simulink model "Signal_Generate_PRN1"  (Simulink 7.3)
settings: Solver=ode45  StartTime=0.0  StopTime=10.0  RelTol=1e-3
values from neighbouring files (symbols this model uses):
  prn = [1 1 1 1 1 1 1 1 1 1 1 1 ... (32736 elements, 32x1023)]    [prn_codes.mat]
libraries: simulink x3, dspswit3 x3, commsynccomp2 x2
settings Model: Creator=xiruizhifu  LastModifiedBy=xiruizhifu
settings SimEventsCC: propDiagAttribOutput=1  propDiagFcnCallOutput=1  propDiagStatOutput=0

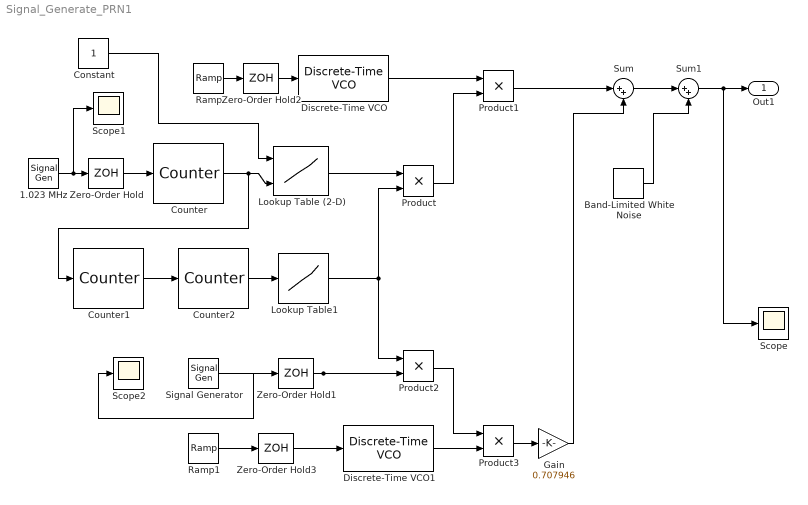
== system Signal_Generate_PRN1 ==
  1.023 MHz : SignalGenerator  WaveForm=square  Frequency=1023000
  Band-Limited White Noise : simulink/Sources/Band-Limited White Noise  SystemSampleTime=-1  Cov=[0.1]  Ts=0.1  seed=[23341]
  Constant : Constant  OutDataType=fixdt(1, 16)  OutScaling=2^0
  Counter : dspswit3/Counter  Direction=Up  CountEvent=Falling edge  CounterSize=User defined  MaxCount=1022  InitialCount=233  Output=Count  HitValue=32  ResetInput=off  SamplesPerFrame=1  Ts=1  CntDtype=double  HitDtype=Logical
  Counter1 : dspswit3/Counter  Direction=Up  CountEvent=Falling edge  CounterSize=User defined  MaxCount=20  InitialCount=0  Output=Count  HitValue=32  ResetInput=off  SamplesPerFrame=1  Ts=1  CntDtype=double  HitDtype=Logical
  Counter2 : dspswit3/Counter  Direction=Up  CountEvent=Falling edge  CounterSize=User defined  MaxCount=1500  InitialCount=0  Output=Count  HitValue=32  ResetInput=off  SamplesPerFrame=1  Ts=1  CntDtype=double  HitDtype=Logical
  Discrete-Time VCO : commsynccomp2/Discrete-Time VCO  SystemSampleTime=-1  Ac=1  Fc=1575420000  Kc=1  Ph=0  ts=0.01
  Discrete-Time VCO1 : commsynccomp2/Discrete-Time VCO  SystemSampleTime=-1  Ac=1  Fc=1575420000  Kc=1  Ph=0.5*pi  ts=0.01
  Gain : Gain  Gain=0.707946  ParameterDataType=fixdt(1, 16)  ParameterScaling=2^0  OutDataType=fixdt(1, 16)  OutScaling=2^0
  Lookup Table (2-D) : Lookup2D  RowIndex=[1:32]  ColumnIndex=[1:1023]  Table=prn  OutDataType=fixdt(1, 16)  OutScaling=2^0
  Lookup Table1 : Lookup  InputValues=[0:1499]  Table=ones(1,1500)  OutDataType=fixdt(1, 16)  OutScaling=2^0
  Product{,1..3} (4 alike) : Product  OutDataType=fixdt(1, 16)  OutScaling=2^0  RndMeth=Zero
  Ramp : simulink/Sources/Ramp  SystemSampleTime=-1  slope=0  start=0  X0=0
  Ramp1 : simulink/Sources/Ramp  SystemSampleTime=-1  slope=0  start=0  X0=0
  Scope : Scope
  Scope1 : Scope
  Scope2 : Scope
      settings: SaveName=ScopeData2
  Signal Generator : SignalGenerator  WaveForm=square  Frequency=10230000
  Sum : Sum  Inputs=|++  OutDataType=fixdt(1, 16)  OutScaling=2^0
  Sum1 : Sum  Inputs=|++  OutDataType=fixdt(1, 16)  OutScaling=2^0
  Zero-Order Hold{,1..3} (4 alike) : ZeroOrderHold
  Out1 : Outport  OutDataType=fixdt(1, 16)  OutScaling=2^0
  wires:
  Counter/1 -> Counter1/1, Lookup Table (2-D)/2
  Lookup Table (2-D)/1 -> Product/1
  Ramp/1 -> Zero-Order Hold2/1
  Discrete-Time VCO/1 -> Product1/1
  Product/1 -> Product1/2
  Counter1/1 -> Counter2/1
  Counter2/1 -> Lookup Table1/1
  Lookup Table1/1 -> Product/2, Product2/1
  Signal Generator/1 -> Zero-Order Hold1/1
  Ramp1/1 -> Zero-Order Hold3/1
  Discrete-Time VCO1/1 -> Product3/2
  Product2/1 -> Product3/1
  Product3/1 -> Gain/1
  Product1/1 -> Sum/1
  Gain/1 -> Sum/2
  Band-Limited White Noise/1 -> Sum1/2
  Constant/1 -> Lookup Table (2-D)/1
  1.023 MHz/1 -> Zero-Order Hold/1, Scope1/1
  Zero-Order Hold/1 -> Counter/1
  Zero-Order Hold1/1 -> Product2/2, Scope2/1
  Zero-Order Hold2/1 -> Discrete-Time VCO/1
  Zero-Order Hold3/1 -> Discrete-Time VCO1/1
  Sum/1 -> Sum1/1
  Sum1/1 -> Out1/1, Scope/1
